simulink model "SingleLinkManipulator"  (R2021a)
settings: Solver=ode14x  StartTime=0.0  StopTime=10.0  RelTol=1e-3
model workspace (MAT data in the model file):
  g = 9.8
  l = 1
  mass = 3
  nu = 6
values from neighbouring files (symbols this model uses):
  x1 = 0    [main.m]    (also in nlcon.m = x(1,b); obj_fun.m = x(1,b))
  x2 = 0    [main.m]    (also in nlcon.m = x(2,b); obj_fun.m = x(2,b))
settings Model: Creator=adekoyoa  LastModifiedBy=adekoyoa

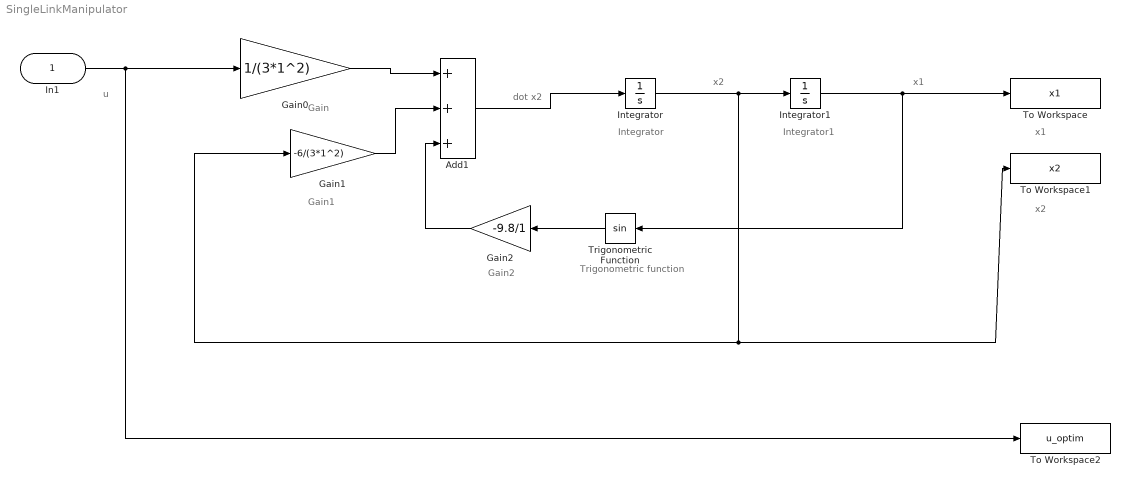
== system SingleLinkManipulator ==
  note: u
  note: Gain2
  note: Trigonometric function
  note: Gain1
  note: Gain
  note: Integrator
  note: Integrator1
  note: x1
  note: x2
  note: dot x2
  note: x2
  note: x1
  In1 : Inport
  Add1 : Sum  Inputs=+++
  Gain0 : Gain  Gain=1/(3*1^2)
  Gain1 : Gain  Gain=-6/(3*1^2)
  Gain2 : Gain  Gain=-9.8/1
  Integrator : Integrator  InitialCondition=x2
  Integrator1 : Integrator  InitialCondition=x1
  To Workspace : ToWorkspace  VariableName=x1  SampleTime=-1
  To Workspace1 : ToWorkspace  VariableName=x2  SampleTime=-1
  To Workspace2 : ToWorkspace  VariableName=u_optim  SampleTime=-1
  Trigonometric Function : Trigonometry
  wires:
  In1/1 -> To Workspace2/1, Gain0/1
  Gain0/1 -> Add1/1
  Gain1/1 -> Add1/2
  Gain2/1 -> Add1/3
  Add1/1 -> Integrator/1
  Integrator/1 -> Gain1/1, To Workspace1/1, Integrator1/1
  Integrator1/1 -> To Workspace/1, Trigonometric Function/1
  Trigonometric Function/1 -> Gain2/1
